simulink model "simulation_sim"  (R2021b)
settings: Solver=VariableStepAuto  StartTime=0.0  StopTime=30.0  RelTol=1e-3
values from neighbouring files (symbols this model uses):
  a = 5    [simulation.m]
  b = 16    [simulation.m]
  c = 3    [simulation.m]
  du = 1    [simulation.m]
  k = 2    [simulation.m]
  step_time = 1    [simulation.m]
  u0 = 0    [simulation.m]
  x0 = 0    [simulation.m]
  x10 = 0    [simulation.m]
settings Model: Creator=rober  LastModifiedBy=rober

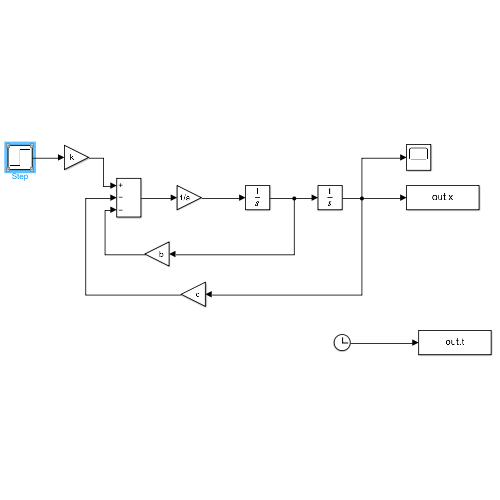
[thumbnail: Simulink's stored preview of the top-level diagram]
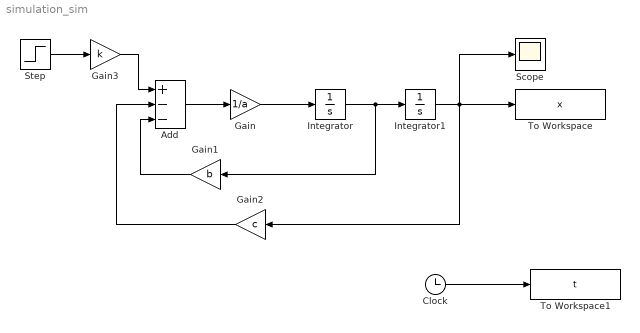
== system simulation_sim ==
  Add : Sum  Inputs=+--
  Clock : Clock
  Gain : Gain  Gain=1/a
  Gain1 : Gain  Gain=b
  Gain2 : Gain  Gain=c
  Gain3 : Gain  Gain=k
  Integrator : Integrator  InitialCondition=x10
  Integrator1 : Integrator  InitialCondition=x0
  Scope : Scope
  Step : Step  Time=step_time  Before=u0  After=u0+du  SampleTime=0
  To Workspace : ToWorkspace  VariableName=x  SampleTime=-1
  To Workspace1 : ToWorkspace  VariableName=t  SampleTime=-1
  wires:
  Integrator/1 -> Gain1/1, Integrator1/1
  Gain/1 -> Integrator/1
  Integrator1/1 -> Gain2/1, Scope/1, To Workspace/1
  Add/1 -> Gain/1
  Gain1/1 -> Add/3
  Gain2/1 -> Add/2
  Gain3/1 -> Add/1
  Step/1 -> Gain3/1
  Clock/1 -> To Workspace1/1
